simulink subsystem "Transaxle"  (R2021a)
settings: Solver=VariableStepAuto  StartTime=0.0  StopTime=10.0  RelTol=1e-3
values from neighbouring files (symbols this model uses):
  igi0 = 7.0518    [loadVariables.m]
  rd = 0.325    [loadVariables.m]
  TransaxleEff = 0.859    [loadVariables.m]
libraries: simulink x1
settings Model: Creator=brand  LastModifiedBy=Brandon

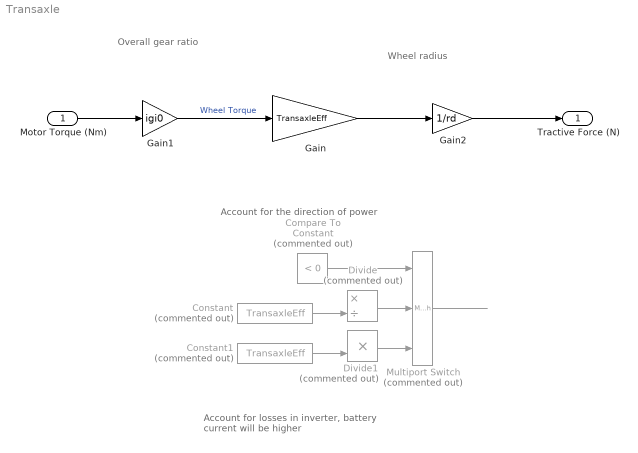
== system Transaxle ==
  note: Wheel radius
  note: Overall gear ratio
  note: Account for the direction of power
  note: Account for losses in inverter, battery current will be higher
  Motor Torque (Nm) : Inport
  Compare To Constant : simulink/Logic and Bit Operations/Compare To Constant  Commented=on  relop=<  const=0  OutDataTypeStr=boolean
  Constant : Constant  Commented=on  Value=TransaxleEff
  Constant1 : Constant  Commented=on  Value=TransaxleEff
  Divide : Product  Commented=on  Inputs=*/
  Divide1 : Product  Commented=on  Inputs=**
  Gain : Gain  Gain=TransaxleEff
  Gain1 : Gain  Gain=igi0
  Gain2 : Gain  Gain=1/rd
  Multiport Switch : MultiPortSwitch  Commented=on  DataPortOrder=Zero-based contiguous  Inputs=2  zeroidx=on
  Tractive Force (N) : Outport
  wires:
  Motor Torque (Nm)/1 -> Gain1/1
  Gain2/1 -> Tractive Force (N)/1
  Divide1/1 -> Multiport Switch/3
  Compare To Constant/1 -> Multiport Switch/1
  Divide/1 -> Multiport Switch/2
  Multiport Switch/1 -> ?
  Constant/1 -> Divide/2
  Constant1/1 -> Divide1/2
  ? -> Divide/1, Divide1/1, Compare To Constant/1  "Wheel Torque"
  Gain1/1 -> Gain/1  "Wheel Torque"
  Gain/1 -> Gain2/1
